simulink model "Lecture13_PolePlacement"  (R2020b)
settings: Solver=VariableStepAuto  StartTime=0.0  StopTime=30  RelTol=1e-3
values from neighbouring files (symbols this model uses):
  Gs = tf([10], [1 2 1])    [Lecture13_PolePlacement.m]    (also in Lecture13_StepResponse.m = tf(Gs_num, Gs_den))
  Kd = 1/2    (= 0.5)    [Assignment3.m]    (also in Lecture13_PolePlacement.m = -0.05; Lecture4_DiscretePID.m = 0.3)
  Ki = kp/ti    [Assignment2.m]    (also in Assignment3.m = 0.5; Assignment4.m = -K(3); Lecture13_PolePlacement.m = 0.0125; Lecture4_DiscretePID.m = 0.8)
  Kp = kp/2    [Assignment2.m]    (also in Assignment3.m = 0.5; Lecture13_PolePlacement.m = -0.025; Lecture4_DiscretePID.m = 0.8)
settings Model: Creator=sebastian  LastModifiedBy=sebastian

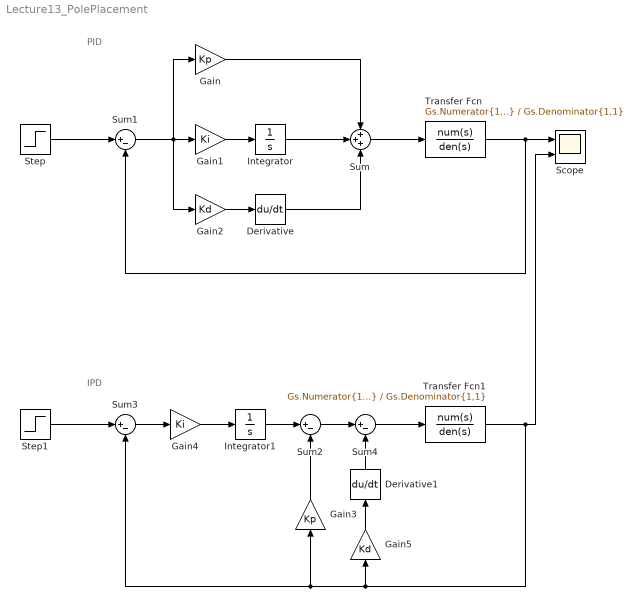
== system Lecture13_PolePlacement ==
  note: PID
  note: IPD
  Derivative : Derivative
  Derivative1 : Derivative
  Gain : Gain  Gain=Kp
  Gain1 : Gain  Gain=Ki
  Gain2 : Gain  Gain=Kd
  Gain3 : Gain  Gain=Kp
  Gain4 : Gain  Gain=Ki
  Gain5 : Gain  Gain=Kd
  Integrator : Integrator
  Integrator1 : Integrator
  Scope : Scope  NumInputPorts=2
  Step : Step  SampleTime=0
  Step1 : Step  SampleTime=0
  Sum : Sum  Inputs=+++
  Sum{1..4} (4 alike) : Sum  Inputs=|+-
  Transfer Fcn : TransferFcn  Numerator=Gs.Numerator{1,1}  Denominator=Gs.Denominator{1,1}
  Transfer Fcn1 : TransferFcn  Numerator=Gs.Numerator{1,1}  Denominator=Gs.Denominator{1,1}
  wires:
  Gain/1 -> Sum/1
  Gain1/1 -> Integrator/1
  Integrator/1 -> Sum/2
  Gain2/1 -> Derivative/1
  Derivative/1 -> Sum/3
  Sum/1 -> Transfer Fcn/1
  Transfer Fcn/1 -> Sum1/2, Scope/1
  Step/1 -> Sum1/1
  Sum1/1 -> Gain2/1, Gain1/1, Gain/1
  Sum3/1 -> Gain4/1
  Step1/1 -> Sum3/1
  Gain5/1 -> Derivative1/1
  Transfer Fcn1/1 -> Gain5/1, Gain3/1, Sum3/2, Scope/2
  Gain4/1 -> Integrator1/1
  Gain3/1 -> Sum2/2
  Derivative1/1 -> Sum4/2
  Integrator1/1 -> Sum2/1
  Sum2/1 -> Sum4/1
  Sum4/1 -> Transfer Fcn1/1
